simulink model "condenser"  (R2021b)
settings: Solver=VariableStepAuto  StartTime=0.0  StopTime=10.0  RelTol=1e-3
settings Model: Creator=Edwar  LastModifiedBy=Edwar

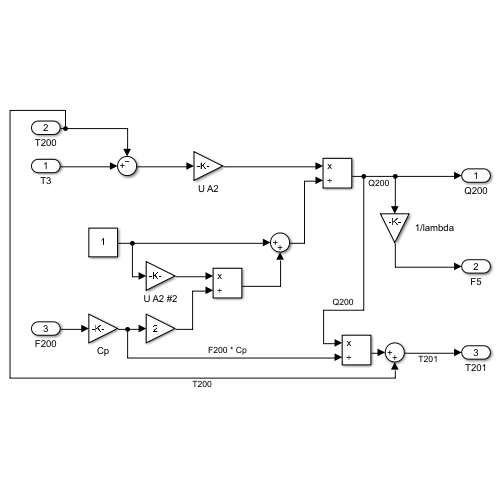
[thumbnail: Simulink's stored preview of the top-level diagram]
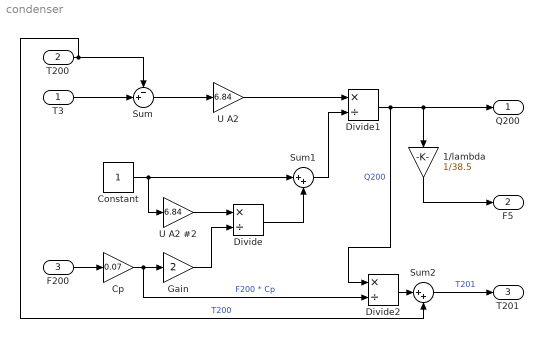
== system condenser ==
  T3 : Inport
  T200 : Inport  Port=2
  F200 : Inport  Port=3
  1/lambda : Gain  Gain=1/38.5
  Constant : Constant
  Cp : Gain  Gain=0.07
  Divide : Product  Inputs=*/
  Divide1 : Product  Inputs=*/
  Divide2 : Product  Inputs=*/
  Gain : Gain  Gain=2
  Sum : Sum  Inputs=-+|
  Sum1 : Sum  Inputs=|++
  Sum2 : Sum  Inputs=|++
  U A2 : Gain  Gain=6.84
  U A2 #2 : Gain  Gain=6.84
  Q200 : Outport
  F5 : Outport  Port=2
  T201 : Outport  Port=3
  wires:
  Sum/1 -> U A2/1
  Constant/1 -> U A2 #2/1, Sum1/1
  Gain/1 -> Divide/2
  U A2 #2/1 -> Divide/1
  Divide/1 -> Sum1/2
  U A2/1 -> Divide1/1
  Sum1/1 -> Divide1/2
  Divide1/1 -> Divide2/1, 1/lambda/1, Q200/1  "Q200"
  T3/1 -> Sum/2
  T200/1 -> Sum2/2, Sum/1  "T200"
  Cp/1 -> Divide2/2, Gain/1  "F200 * Cp"
  F200/1 -> Cp/1
  Divide2/1 -> Sum2/1
  Sum2/1 -> T201/1  "T201"
  1/lambda/1 -> F5/1
